simulink subsystem "SteeringSystem"  (R2023b)
settings: Solver=VariableStepAuto  StartTime=0.0  StopTime=10.0  RelTol=1e-3
undefined symbols (not defined in the file): PlntVehTrckWdth
libraries: vehdynlibsteering x2
settings Model: ModifiedByFormat=The MathWorks, Inc.  Creator=The MathWorks, Inc.  LastModifiedBy=The MathWorks, Inc.
settings OptimizationCC: ReuseModelBlockBuffer=off

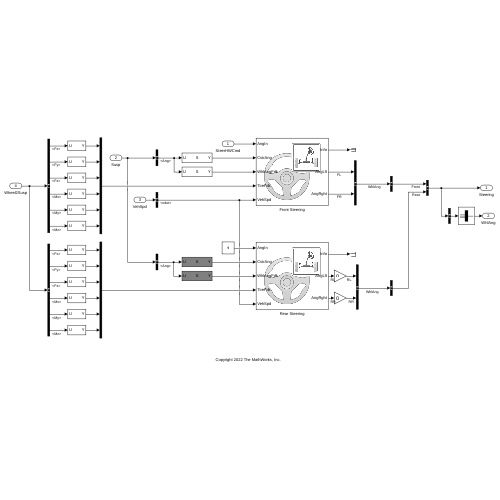
[thumbnail: Simulink's stored preview of the top-level diagram]
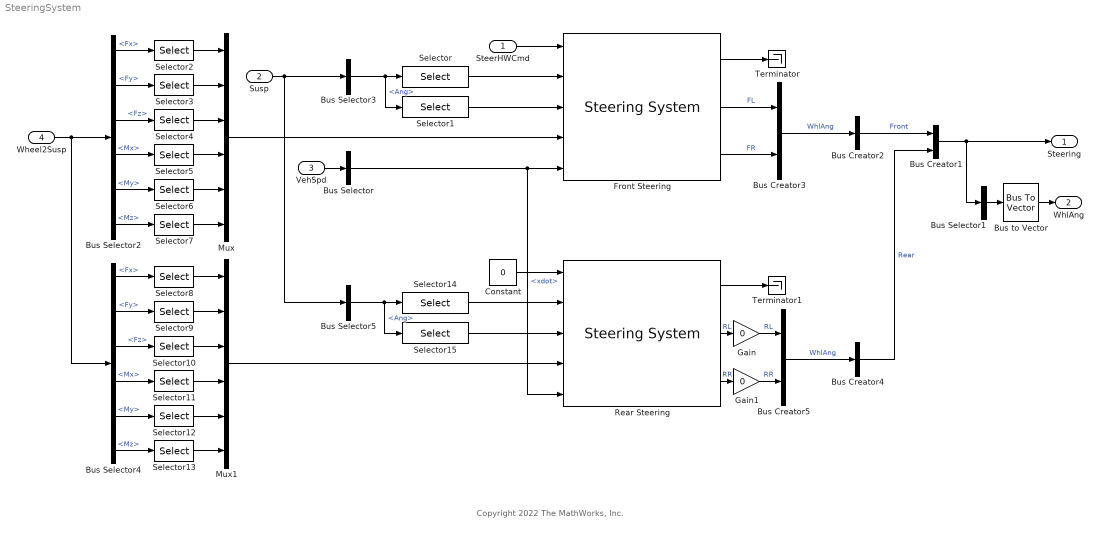
== system SteeringSystem ==
  note: Copyright 2022 The MathWorks, Inc.
  SteerHWCmd : Inport
  Susp : Inport  Port=2
  VehSpd : Inport  Port=3
  Wheel2Susp : Inport  Port=4
  Bus Creator1 : BusCreator  Inputs=2
  Bus Creator2 : BusCreator  Inputs=1
  Bus Creator3 : BusCreator  Inputs=2
  Bus Creator4 : BusCreator  Inputs=1
  Bus Creator5 : BusCreator  Inputs=2
  Bus Selector : BusSelector  OutputSignals=BdyFrm.Cg.Vel.xdot
  Bus Selector1 : BusSelector  OutputSignals=Front.WhlAng.FL,Front.WhlAng.FR,Rear.WhlAng.RL,Rear.WhlAng.RR  OutputAsBus=on
  Bus Selector2 : BusSelector  OutputSignals=SuspFrame.Fx,SuspFrame.Fy,SuspFrame.Fz,SuspFrame.Mx,SuspFrame.My,SuspFrame.Mz
  Bus Selector3 : BusSelector  OutputSignals=SuspChassis.Whl.Ang
  Bus Selector4 : BusSelector  OutputSignals=SuspFrame.Fx,SuspFrame.Fy,SuspFrame.Fz,SuspFrame.Mx,SuspFrame.My,SuspFrame.Mz
  Bus Selector5 : BusSelector  OutputSignals=SuspChassis.Whl.Ang
  Bus to Vector : BusToVector
  Constant : Constant  Value=0
  Front Steering : vehdynlibsteering/Steering System  StrgType=Rack and pinion  IntmdShaftType=Single Cardan joint  PwrAst=on  AckStr=on  Dst=PlntSteerDst  PwrAstOverride=off  AckStrOverride=off  KingpinOverride=off  Loc=Front  StrIn=Angle  TrckWdth=PlntVehTrckWdth(1)  StrRng=PlntSteerRange  DbWdth=0  StrWhlInert=PlntSteerUpperInertia  StrColInert=PlntSteerLowerInertia  KngpnOfst=PlntSteerKngpnOfst  Lambda=PlntSteerLambda  HbLead=PlntSteerHbLead  StcLdRadius=PlntSteerStcLdRadius  OvrlStrRatio=PlntSteerRatio  StrgAngBpts="[-6.2832   -5.0265   -3.7699   -2.5133   -1.2566         0    1.2566    2.5133    3.7699    5.0265    6.2832]"  CstrAng=0  StrgRatioType=Constant  RckGn=PlntSteerRckGn  RckGnTbl=ones(1,11)*0.0057*2*pi  RckPnAlgm=Kinematics  RackDispBpts=[-40 -19.2 -4.53 4.53 19.2 40]  RghtWhlAngTbl=[-1.5*pi -0.72*pi -0.17*pi 0.17*pi 0.72*pi 1.5*pi]/13.5  RghtWhlStrSpdTbl=[0.008726624950158,0.008727065906090,0.008727190569212,0.008727190569212,0.008727065906090,0.008726624950158]  LftWhlAngTbl=[-1.5*pi -0.72*pi -0.17*pi 0.17*pi 0.72*pi 1.5*pi]/13.5  LftWhlStrSpdTbl=[0.008726624950158,0.008727065906090,0.008727190569212,0.008727190569212,0.008727065906090,0.008726624950158]  StrgArmLngth=PlntSteerStrgArmLngth  RckCsLngth=PlntSteerRckCsLngth  TieRodLngth=PlntSteerTieRodLngth  D=0.2  Epsilon=PlntSteerEpsilon  PnInert=PlntSteerPnInert  SptlAng=2.6178  Alpha_b=2.6178  Alpha_c=2.7051  Sigma_bc=0.2618  Gamma=0.2618  TrqBpts=PlntSteerWheelTrqBpt  VehSpdBpts=[0 20]  TrqTbl=PlntSteerTrqAsstTbl  TrqLmt=PlntSteerTrqLimit  PwrLmt=PlntSteerPwrLimit  Eta=1  omega_c=PlntSteerWc  AckParamType=Constant  PctAck=PlntSteerPctAck  PctAckTbl=ones(1,11)*100  SlgStf=PlntSteerSlgStf  UpprFric=PlntSteerUpprFric  PrsFric=PlntSteerPrsFric  MaxStf=PlntSteerMaxStf  MaxUpprFric=PlntSteerMaxUpprFric  MaxDamp=PlntSteerMaxDamp  TorStf=PlntSteerTorStf  TorDamp=PlntSteerTorDamp
  Gain : Gain  Gain=0
  Gain1 : Gain  Gain=0
  Mux : Mux  Inputs=6
  Mux1 : Mux  Inputs=6
  Rear Steering : vehdynlibsteering/Steering System  StrgType=Rack and pinion  IntmdShaftType=Single Cardan joint  PwrAst=on  AckStr=on  Dst=PlntSteerDst  PwrAstOverride=off  AckStrOverride=off  KingpinOverride=off  Loc=Rear  StrIn=Angle  TrckWdth=PlntVehTrckWdth(1)  StrRng=PlntSteerRange  DbWdth=0  StrWhlInert=PlntSteerUpperInertia  StrColInert=PlntSteerLowerInertia  KngpnOfst=PlntSteerKngpnOfst  Lambda=PlntSteerLambda  HbLead=PlntSteerHbLead  StcLdRadius=PlntSteerStcLdRadius  OvrlStrRatio=PlntSteerRatio  StrgAngBpts="[-6.2832   -5.0265   -3.7699   -2.5133   -1.2566         0    1.2566    2.5133    3.7699    5.0265    6.2832]"  CstrAng=0  StrgRatioType=Constant  RckGn=PlntSteerRckGn  RckGnTbl=ones(1,11)*0.0057*2*pi  RckPnAlgm=Kinematics  RackDispBpts=[-40 -19.2 -4.53 4.53 19.2 40]  RghtWhlAngTbl=[-1.5*pi -0.72*pi -0.17*pi 0.17*pi 0.72*pi 1.5*pi]/13.5  RghtWhlStrSpdTbl=[0.008726624950158,0.008727065906090,0.008727190569212,0.008727190569212,0.008727065906090,0.008726624950158]  LftWhlAngTbl=[-1.5*pi -0.72*pi -0.17*pi 0.17*pi 0.72*pi 1.5*pi]/13.5  LftWhlStrSpdTbl=[0.008726624950158,0.008727065906090,0.008727190569212,0.008727190569212,0.008727065906090,0.008726624950158]  StrgArmLngth=PlntSteerStrgArmLngth  RckCsLngth=PlntSteerRckCsLngth  TieRodLngth=PlntSteerTieRodLngth  D=0.2  Epsilon=PlntSteerEpsilon  PnInert=PlntSteerPnInert  SptlAng=2.6178  Alpha_b=2.6178  Alpha_c=2.7051  Sigma_bc=0.2618  Gamma=0.2618  TrqBpts=PlntSteerWheelTrqBpt  VehSpdBpts=[0 20]  TrqTbl=PlntSteerTrqAsstTbl  TrqLmt=PlntSteerTrqLimit  PwrLmt=PlntSteerPwrLimit  Eta=1  omega_c=PlntSteerWc  AckParamType=Constant  PctAck=PlntSteerPctAck  PctAckTbl=ones(1,11)*100  SlgStf=PlntSteerSlgStf  UpprFric=PlntSteerUpprFric  PrsFric=PlntSteerPrsFric  MaxStf=PlntSteerMaxStf  MaxUpprFric=PlntSteerMaxUpprFric  MaxDamp=PlntSteerMaxDamp  TorStf=PlntSteerTorStf  TorDamp=PlntSteerTorDamp
  Selector : Selector  NumberOfDimensions=2  InputPortWidth=3  IndexOptions=Index vector (dialog),Index vector (dialog)  Indices=2,[1 2]  OutputSizes=1,1
  Selector1 : Selector  NumberOfDimensions=2  InputPortWidth=3  IndexOptions=Index vector (dialog),Index vector (dialog)  Indices=3,[1 2]  OutputSizes=1,1
  Selector{8..13} (6 alike) : Selector  InputPortWidth=4  IndexOptions=Index vector (dialog)  Indices=[3 4]  OutputSizes=1
  Selector14 : Selector  NumberOfDimensions=2  InputPortWidth=3  IndexOptions=Index vector (dialog),Index vector (dialog)  Indices=2,[1 2]  OutputSizes=1,1
  Selector15 : Selector  NumberOfDimensions=2  InputPortWidth=3  IndexOptions=Index vector (dialog),Index vector (dialog)  Indices=3,[1 2]  OutputSizes=1,1
  Selector{2..7} (6 alike) : Selector  InputPortWidth=4  IndexOptions=Index vector (dialog)  Indices=[1 2]  OutputSizes=1
  Terminator : Terminator
  Terminator1 : Terminator
  Steering : Outport
  WhlAng : Outport  Port=2  Unit=rad  VectorParamsAs1DForOutWhenUnconnected=off
  wires:
  Constant/1 -> Rear Steering/1
  Selector15/1 -> Rear Steering/3
  Selector14/1 -> Rear Steering/2
  Bus Selector5/1 -> Selector15/1, Selector14/1  "<Ang>"
  Selector/1 -> Front Steering/2
  Bus Selector4/5 -> Selector12/1  "<My>"
  Bus Selector4/2 -> Selector9/1  "<Fy>"
  Selector8/1 -> Mux1/1
  Bus Selector4/3 -> Selector10/1  "<Fz>"
  Mux1/1 -> Rear Steering/4
  Bus Selector4/1 -> Selector8/1  "<Fx>"
  Bus Selector4/4 -> Selector11/1  "<Mx>"
  Bus Selector4/6 -> Selector13/1  "<Mz>"
  Wheel2Susp/1 -> Bus Selector2/1, Bus Selector4/1
  Selector11/1 -> Mux1/4
  Selector9/1 -> Mux1/2
  Selector10/1 -> Mux1/3
  Selector13/1 -> Mux1/6
  Selector12/1 -> Mux1/5
  Mux/1 -> Front Steering/4
  Selector7/1 -> Mux/6
  Selector6/1 -> Mux/5
  Selector5/1 -> Mux/4
  Selector4/1 -> Mux/3
  Selector3/1 -> Mux/2
  Selector2/1 -> Mux/1
  Bus Selector2/6 -> Selector7/1  "<Mz>"
  Bus Selector2/5 -> Selector6/1  "<My>"
  Bus Selector2/4 -> Selector5/1  "<Mx>"
  Bus Selector2/3 -> Selector4/1  "<Fz>"
  Bus Selector2/2 -> Selector3/1  "<Fy>"
  Bus Selector2/1 -> Selector2/1  "<Fx>"
  Selector1/1 -> Front Steering/3
  Gain1/1 -> Bus Creator5/2  "RR"
  Rear Steering/2 -> Gain/1  "RL"
  Rear Steering/1 -> Terminator1/1
  Front Steering/1 -> Terminator/1
  Bus Selector/1 -> Front Steering/5, Rear Steering/5  "<xdot>"
  Bus Selector3/1 -> Selector/1, Selector1/1  "<Ang>"
  SteerHWCmd/1 -> Front Steering/1
  Bus to Vector/1 -> WhlAng/1
  Bus Creator1/1 -> Bus Selector1/1, Steering/1
  Bus Selector1/1 -> Bus to Vector/1
  Bus Creator5/1 -> Bus Creator4/1  "WhlAng"
  Front Steering/3 -> Bus Creator3/2  "FR"
  Bus Creator2/1 -> Bus Creator1/1  "Front"
  Rear Steering/3 -> Gain1/1  "RR"
  Gain/1 -> Bus Creator5/1  "RL"
  Front Steering/2 -> Bus Creator3/1  "FL"
  Bus Creator4/1 -> Bus Creator1/2  "Rear"
  Bus Creator3/1 -> Bus Creator2/1  "WhlAng"
  Susp/1 -> Bus Selector3/1, Bus Selector5/1
  VehSpd/1 -> Bus Selector/1
